simulink model "SAMPLE_logicV2"  (R2017a)
settings: Solver=VariableStepAuto  StartTime=0.0  StopTime=inf  RelTol=1e-3
libraries: martin_sean_RoombaLib x6, realtime_pacer_lib x1
settings Model: Creator=Sean  LastModifiedBy=Sean

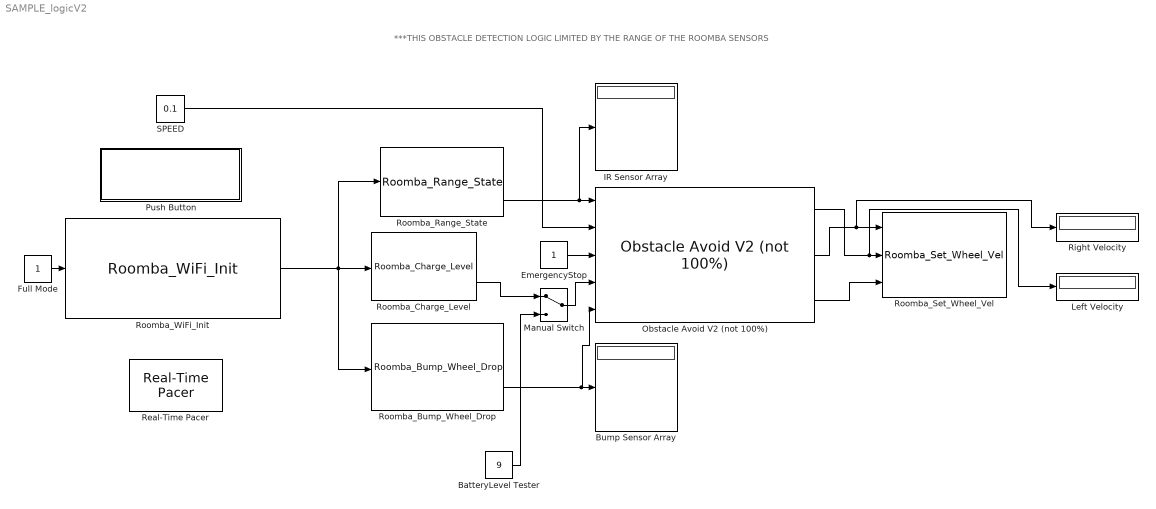
== system SAMPLE_logicV2 ==
  note: ***THIS OBSTACLE DETECTION LOGIC LIMITED BY THE RANGE OF THE ROOMBA SENSORS
  BatteryLevel Tester : Constant  Value=9
  Bump Sensor Array : Display
  EmergencyStop : Constant
  Full Mode : Constant
  IR Sensor Array : Display
  Left Velocity : Display
  Manual Switch : ManualSwitch
  Obstacle Avoid V2 (not 100%) : martin_sean_RoombaLib/Obstacle Avoid V2 (not 100%)  SystemSampleTime=-1
  Push Button : Subsystem  DialogController=hmiCreateDDGDialog  IsWebBlock=on  mask(MWDashboardBlock){webBlockId=329c33c9-0033-425f-9c2b-cdea2ef2ab51, webBlockType=pushbutton, ShowInLibBrwoser=on, ShowInitialText=on, HMISrcModelName=SAMPLE_logicV2}
      mask prompts: webBlockId "WebBlock Id"; webBlockType "WebBlock Type"; HMISrcModelName "Source Model"
      mask help: SimulinkHMI:dialogs:PushButtonDialogDesc
      mask Help: helpview([docroot '/mapfiles/simulink.map'], 'hmi_push_button')
      mask Display:
      | model = bdroot(gcb);
      | if strcmp(get_param(model,'BlockDiagramType'), 'library')
      |     image([(matlabroot) '/toolbox/simulink/hmi/icons/PushButton.png']);
      | end
  Real-Time Pacer : realtime_pacer_lib/Real-Time Pacer  simTimePerRealTime=1
  Right Velocity : Display
  Roomba_Bump_Wheel_Drop : martin_sean_RoombaLib/Roomba_Bump_Wheel_Drop
  Roomba_Charge_Level : martin_sean_RoombaLib/Roomba_Charge_Level  Description=Returns the battery charge level on the Roomba as a percentage. Updates every 100 seconds.
  Roomba_Range_State : martin_sean_RoombaLib/Roomba_Range_State  Description=|
      | Returns [1x6] array containing the state of the six IR sensors on the front of the Roomba. A 
      | '1' indicates there is an object ahead and a '0' indicates no object.
  Roomba_Set_Wheel_Vel : martin_sean_RoombaLib/Roomba_Set_Wheel_Vel  Description=|
      | Sets the right and left wheel velocities on the Roomba. The values are in meters/sec between 
      | [-0.5, 0.5]. Negative velocity is backwards.
  Roomba_WiFi_Init : martin_sean_RoombaLib/Roomba_WiFi_Init  Description=|  Priority=-1000
      | Initializes a WiFi connection to the Roomba. The RooWiFi module is used. Takes the mode as an
      | input. For instance, Mode = 1 will set up a connection to the Roomba over RooWiFi on 10.0.0.1
      | and place it in 'full' mode.
      | 
      | A 0 is returned after successful initialization.
      | 
      | RooWiFi documentation:
      | http://www.roowifi.com/wp-content/uploads/RwRemote_User_Guide_v2_rev15.pdf
  SPEED : Constant  Value=0.1
  wires:
  EmergencyStop/1 -> Obstacle Avoid V2 (not 100%)/3
  Roomba_WiFi_Init/1 -> Roomba_Bump_Wheel_Drop/1, Roomba_Range_State/1, Roomba_Charge_Level/1
  SPEED/1 -> Obstacle Avoid V2 (not 100%)/2
  Manual Switch/1 -> Obstacle Avoid V2 (not 100%)/4
  Roomba_Bump_Wheel_Drop/2 -> Obstacle Avoid V2 (not 100%)/5, Bump Sensor Array/1
  BatteryLevel Tester/1 -> Manual Switch/2
  Roomba_Range_State/2 -> Obstacle Avoid V2 (not 100%)/1, IR Sensor Array/1
  Full Mode/1 -> Roomba_WiFi_Init/1
  Roomba_Charge_Level/2 -> Manual Switch/1
  Obstacle Avoid V2 (not 100%)/1 -> Left Velocity/1, Roomba_Set_Wheel_Vel/2
  Obstacle Avoid V2 (not 100%)/2 -> Roomba_Set_Wheel_Vel/1, Right Velocity/1
  Obstacle Avoid V2 (not 100%)/3 -> Roomba_Set_Wheel_Vel/3

== system SAMPLE_logicV2/Push Button ==
